simulink model "BD12"  (R2014a)
settings: Solver=ode45  StartTime=0.0  StopTime=10.0  RelTol=1e-3
settings Model: Creator=Usman Arshad  LastModifiedBy=Usman Arshad

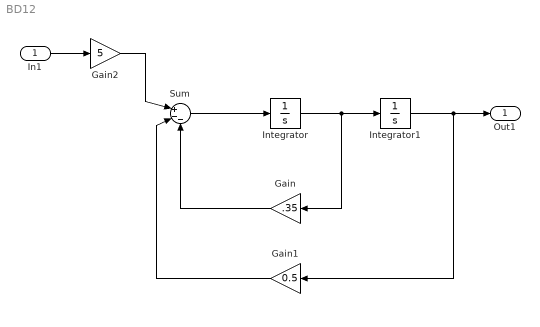
== system BD12 ==
  In1 : Inport
  Gain : Gain  Gain=.35
  Gain1 : Gain  Gain=0.5
  Gain2 : Gain  Gain=5
  Integrator : Integrator
  Integrator1 : Integrator
  Sum : Sum  Inputs=|+--
  Out1 : Outport
  wires:
  Gain/1 -> Sum/3
  Gain1/1 -> Sum/2
  Sum/1 -> Integrator/1
  Integrator/1 -> Gain/1, Integrator1/1
  In1/1 -> Gain2/1
  Gain2/1 -> Sum/1
  Integrator1/1 -> Gain1/1, Out1/1
